simulink model "planner_contral"  (R2023b)
settings: Solver=FixedStepAuto  StartTime=0  StopTime=inf  FixedStep=0.001  RelTol=1e-3
undefined symbols (not defined in the file): aubr, c_factor, cf, cr, iniObsHeading1, iniObsHeading2, iniObsPos1, iniObsPos2, KD_PID_distance, KD_PID_speed, KI_PID_distance, KI_PID_speed, KP_PID_distance, KP_PID_speed, la, lb, LQR_K1, LQR_K2, LQR_K3, LQR_K4, m, rack_displacement, refInfo_obs1, refInfo_obs2, right_wheel_ground, rightWaypoints, tablebr, vubr, vx_break_point
libraries: Solver_SF x1
(part 8 of 8)

== matlab function planner_contral/Subsystem5/packaging ==
  data: dynamic_obs1_x input; obs_x_set_gcs output; dynamic_obs1_y input; dynamic_obs1_heading input; dynamic_obs1_speed input; dynamic_obs2_x input; dynamic_obs2_y input; dynamic_obs2_heading input; obs_y_set_gcs output; obs_velocity_set_gcs output; obs_heading_set_gcs output; dynamic_obs2_speed input; stactic_obs1_x input; stactic_obs1_y input; stactic_obs1_heading input; stactic_obs1_speed input; stactic_obs2_x input; stactic_obs2_y input; stactic_obs2_heading input; stactic_obs2_speed input
function [obs_x_set_gcs,obs_y_set_gcs,obs_velocity_set_gcs,obs_heading_set_gcs] = ...
    fcn(dynamic_obs1_x,dynamic_obs1_y,dynamic_obs1_heading,dynamic_obs1_speed,...
    dynamic_obs2_x,dynamic_obs2_y,dynamic_obs2_heading,dynamic_obs2_speed,...
    stactic_obs1_x,stactic_obs1_y,stactic_obs1_heading,stactic_obs1_speed,...
    stactic_obs2_x,stactic_obs2_y,stactic_obs2_heading,stactic_obs2_speed)
%gcs 全局坐标系global coordinate system
%该函数是感知模块，输出障碍物的位置，速度大小，速度方向与世界坐标系x轴的夹角
%输入：定位信息host_x,host_y,host_heading_xy 世界坐标系
%      障碍物在传感器坐标系下的极坐标range，theta
%      障碍物的速度大小 velocity
%      障碍物的速度方向与x轴的夹角 heading
%输出：障碍物在世界坐标系下的坐标 x y v v与x轴的夹角heading
%      注意输出的heading是障碍物的速度heading，不是障碍物的几何heading

%传感器最多输出32个障碍物信息，但是事先不知道有多少个障碍物，所以要做个缓冲

%输出初始化
obs_x_set_gcs = ones(32,1)*nan;
obs_y_set_gcs = ones(32,1)*nan;
obs_velocity_set_gcs = ones(32,1)*nan;
obs_heading_set_gcs = ones(32,1)*nan;
%传感器极坐标的角度顺时针为正，世界坐标是逆时针为正


%计算障碍物的世界坐标

% ===== 1) dynamic obstacle 1 =====
obs_x_set_gcs(1) = dynamic_obs1_x;
obs_y_set_gcs(1) = dynamic_obs1_y;
obs_heading_set_gcs(1) = dynamic_obs1_heading;
obs_velocity_set_gcs(1) = dynamic_obs1_speed;

% ===== 2) dynamic obstacle 2 =====
obs_x_set_gcs(2) = dynamic_obs2_x;
obs_y_set_gcs(2) = dynamic_obs2_y;
obs_heading_set_gcs(2) = dynamic_obs2_heading;
obs_velocity_set_gcs(2) = dynamic_obs2_speed;

% ===== 3) static obstacle 1 =====
obs_x_set_gcs(3) = stactic_obs1_x;
obs_y_set_gcs(3) = stactic_obs1_y;
obs_heading_set_gcs(3) = stactic_obs1_heading;
obs_velocity_set_gcs(3) = stactic_obs1_speed;

% ===== 4) static obstacle 2 =====
obs_x_set_gcs(4) = stactic_obs2_x;
obs_y_set_gcs(4) = stactic_obs2_y;
obs_heading_set_gcs(4) = stactic_obs2_heading;
obs_velocity_set_gcs(4) = stactic_obs2_speed;

== matlab function planner_contral/decision_planning/EMplanner/path decision task/increase DP path nodes ==
  data: dp_path_s_init input; dp_path_s_final output; dp_path_l_init input; plan_start_s input; plan_start_l input; plan_start_dl input; plan_start_ddl input; dp_path_l_final output; dp_path_dl_final output; dp_path_ddl_final output
function [dp_path_s_final,dp_path_l_final,dp_path_dl_final,dp_path_ddl_final] = ...
    fcn(dp_path_s_init,dp_path_l_init,plan_start_s,plan_start_l,plan_start_dl,plan_start_ddl)
% 该函数将增密dp_path_s,dp_path_l
% 由于事先不知道动态规划采样的行和列，也就不知道动态规划计算的曲线有多长，因此需要做缓冲
% 每1“米”采样一个点，一共采60个
ds = 1;
% 输出初始化
dp_path_s_final = ones(60,1)*nan;
dp_path_l_final = ones(60,1)*nan;
dp_path_dl_final = ones(60,1)*nan;
dp_path_ddl_final = ones(60,1)*nan;

% 设置五次多项式的起点
start_s = plan_start_s;
start_l = plan_start_l;
start_dl = plan_start_dl;
start_ddl = plan_start_ddl;

s_cur = [];
l_temp = [];
dl_temp =[];
ddl_temp = [];

for i = 1:length(dp_path_s_init)
    if dp_path_s_init(i) == -1
        break;
    end
    for j = 1:10000
        %采样s
        s_node = start_s + ds*(j - 1);
        if s_node < dp_path_s_init(i)
            s_cur = [s_cur,s_node];
        else
            break;
        end
    end
    end_s = dp_path_s_init(i);
    end_l = dp_path_l_init(i);
    end_dl = 0;
    end_ddl = 0;
    coeff = CalcQuinticCoeffient(start_l,start_dl,start_ddl,end_l,end_dl,end_ddl,start_s,end_s);
    a0 = coeff(1);
    a1 = coeff(2);
    a2 = coeff(3);
    a3 = coeff(4);
    a4 = coeff(5);
    a5 = coeff(6);
    l = a0 * ones(1,length(s_cur)) + a1 * s_cur + a2 * s_cur.^2 + a3 * s_cur.^3 +...
        a4 * s_cur.^4 + a5 * s_cur.^5;
    dl = a1 * ones(1,length(s_cur)) + 2 * a2 * s_cur + 3 * a3 * s_cur.^2 + ...
        4 * a4 * s_cur.^3 + 5 * a5 * s_cur.^4;
    ddl = 2 * a2 * ones(1,length(s_cur)) + 6 * a3 * s_cur + 12 * a4 * s_cur.^2 + ...
        20 * a5 * s_cur.^3;
    % 把 l dl ddl 的结果保存
    l_temp = [l_temp,l];
    dl_temp = [dl_temp,dl];
    ddl_temp = [ddl_temp,ddl];
    % end的值赋值给start 做下一步循环
    start_s = end_s;
    start_l = end_l;
    start_dl = end_dl;
    start_ddl = end_ddl;
    s_cur = [];
end
   for k = 1:length(l_temp)
       if k == 61
           break;
       end
       dp_path_s_final(k) = plan_start_s + ds * (k - 1);
       dp_path_l_final(k) = l_temp(k);
       dp_path_dl_final(k) = dl_temp(k);
       dp_path_ddl_final(k) = ddl_temp(k);
   end
end

function coeff = CalcQuinticCoeffient(start_l,start_dl,start_ddl,end_l,end_dl,end_ddl,start_s,end_s)
    % l = a0 + a1*s + a2*s^2 + a3*s^3 + a4*s^4 + a5*s^5
    % l' = a1 + 2 * a2 * s + 3 * a3 * s^2 + 4 * a4 * s^3 + 5 * a5 * s^4
    % l'' = 2 * a2 + 6 * a3 * s + 12 * a4 * s^2 + 20 * a5 * s^3
    start_s2 = start_s * start_s;
    start_s3 = start_s2 * start_s;
    start_s4 = start_s3 * start_s;
    start_s5 = start_s4 * start_s;
    end_s2 = end_s * end_s;
    end_s3 = end_s2 * end_s;
    end_s4 = end_s3 * end_s;
    end_s5 = end_s4 * end_s;
    A = [1,start_s, start_s2,     start_s3,     start_s4,      start_s5;
         0 1,       2 * start_s,  3 * start_s2, 4 * start_s3,  5 * start_s4;
         0 0,       2,            6 * start_s,  12 * start_s2, 20 * start_s3;
         1,end_s, end_s2,     end_s3,     end_s4,      end_s5;
         0,1,     2 * end_s,  3 * end_s2, 4 * end_s3,  5 * end_s4;
         0,0,     2,          6 * end_s,  12 * end_s2, 20 * end_s3;];
    B = [start_l;
         start_dl;
         start_ddl;
         end_l;
         end_dl;
         end_ddl;];
     coeff = A \ B;
    
end

== matlab function planner_contral/decision_planning/EMplanner/path decision task/path decision with dynamic planning(dp) ==
  data: staticobs_s_set input; dp_path_s output; staticobs_l_set input; staticobs_heading input; plan_start_s input; plan_start_l input; plan_start_dl input; plan_start_dll input; w_cost_collision input; w_cost_smooth_dl input; w_cost_smooth_ddl input; w_cost_smooth_dddl input; w_cost_ref input; row input; col input; sample_s input; sample_l input; dp_path_l output; dynamic_obs_s input; dynamic_obs_l input; dynamic_obs_heading input
function [dp_path_s,dp_path_l] = fcn(staticobs_s_set,staticobs_l_set,staticobs_heading,plan_start_s,plan_start_l,plan_start_dl,...
    plan_start_dll,w_cost_collision,w_cost_smooth_dl,w_cost_smooth_ddl,w_cost_smooth_dddl,w_cost_ref,row,col,sample_s,sample_l,dynamic_obs_s,dynamic_obs_l,dynamic_obs_heading)
%该函数为路径决策算法动态规划的主函数
% 输入：obs s l set 筛选后的障碍物sl信息
%       plan_start s l dl ddl 规划起点信息
%       w_cost_obs,w_cost_smooth_dl,w_cost_smooth_ddl,w_cost_smooth_dddl,w_cost_ref动态规划代价权重
%       row col 动态规划采样点的行数和列数(row必须是奇数，col必须是6)
%       sample_s,sample_l 采样的s l 长度
% 输出：dp_path_l,dp_path_s 动态规划的路径sl,此路径不包含规划起点  

%动态规划最优的数据结构是结构体矩阵，但是simulink不支持结构体矩阵，所以动态规划算法写的相对难以理解

%声明二维矩阵变量node_cost，node_cost(i,j)表示从起点出发，到行i列j节点的最小代价为node_cost(i,j)
node_cost = ones(row,col)*inf;%初始化为无穷大

%声明二维矩阵变量pre_node_index pre_node_index(i,j)表示从起点到行i列j的节点的最优路径中前一个节点的行号为
%pre_node_index(i,j)
%例：比如一条最优路径为 起点 -> node(1,1) -> node(2,2) -> node(3,3)
%则pre_node_index(3,3) = 2 (最优路径的前一个节点是node(2,2) 取它的行号）
%  pre_node_index(2,2) = 1 (最优路径的前一个节点是node(1,1) 取它的行号）
%  pre_node_index(1,1) = 0 (起点的行号默认是0)

% 其实pre_node_index就是当找到最小代价的路径后从终点到起点反向选择出最优路径的
%如果用结构体矩阵完全没有必要弄得这么麻烦，但是simulink不支持
pre_node_index = zeros(row,col);%初始化，所有节点的上个最优节点的行号都是0，也就是起点

%先计算从起点到第一列的cost
for i = 1:row
    node_cost(i,1) = CalcStartCost(plan_start_s,plan_start_l,plan_start_dl,...
    plan_start_dll,i,sample_s,sample_l,w_cost_collision,w_cost_smooth_dl,...
    w_cost_smooth_ddl,w_cost_smooth_dddl,w_cost_ref,staticobs_s_set,staticobs_l_set,staticobs_heading,row)+ CalcStartCost(plan_start_s,plan_start_l,plan_start_dl,...
    plan_start_dll,i,sample_s,sample_l,w_cost_collision,w_cost_smooth_dl,...
    w_cost_smooth_ddl,w_cost_smooth_dddl,w_cost_ref,dynamic_obs_s,dynamic_obs_l,dynamic_obs_heading,row);
end
% 动态规划主函数，从第二列开始
for j = 2:col
    for i = 1:row
        %计算当前node(i,j)的s l
        cur_node_s = plan_start_s + j * sample_s;
        cur_node_l = ((row + 1)/2 - i) * sample_l;
        %遍历前一列的节点
        for k = 1:row
            %计算前一列节点的s l
            pre_node_s = plan_start_s + (j - 1) * sample_s;
            pre_node_l = ((row + 1)/2 - k) * sample_l;
            cost_neighbour = CalcNeighbourCost(pre_node_s,pre_node_l,cur_node_s,cur_node_l,w_cost_collision,...
    w_cost_smooth_dl,w_cost_smooth_ddl,w_cost_smooth_dddl,w_cost_ref,staticobs_s_set,staticobs_l_set,staticobs_heading)+ CalcNeighbourCost(pre_node_s,pre_node_l,cur_node_s,cur_node_l,w_cost_collision,...
    w_cost_smooth_dl,w_cost_smooth_ddl,w_cost_smooth_dddl,w_cost_ref,dynamic_obs_s,dynamic_obs_l,dynamic_obs_heading);
            %起点到上一个节点的最小代价为node_cost(k,j-1)
            pre_min_cost = node_cost(k,j-1);
            %起点到node_cost(i,j)的最小代价 为node_cost(k,j-1)
            %再加上node(k,j-1)到node(i,j)的代价 (k = 1,2,3,4...row) 中最小的
            cost_temp = pre_min_cost + cost_neighbour;
            if cost_temp < node_cost(i,j)
                node_cost(i,j) = cost_temp;
                %把最优路径上一列节点的行号记录下来
                pre_node_index(i,j) = k;
            end
        end      
    end
end
%找到node_cost最后一列中，cost最小的，记代价最小的行号为index
index = 0;
min_cost = inf;
for i = 1:row
    if node_cost(i,end) < min_cost
        min_cost = node_cost(i,end);
        index = i;
    end
end
%动态规划最优路径初始化
dp_node_list_row = zeros(col,1);
%从后往前逆推
cur_index = index;
for i = 1:col
    %记录cur_index前面节点的行号
    pre_index = pre_node_index(cur_index,end - i + 1);
    %把cur_index放到dp_node_list_row对应的位置
    dp_node_list_row(col - i + 1) = cur_index;
    %再把pre_index 赋给 cur_index 进行下一步递推
    cur_index = pre_index;
end
% 输出初始化，由于事先不知道横纵向的采样列数，因此需要做缓冲，横纵向采样的列数不就是固定下来的吗？？？笑话
dp_path_s = ones(15,1)*-1;
dp_path_l = ones(15,1)*-1;
for i = 1:col  %最多到col，其余均为-1；
    dp_path_s(i) = plan_start_s + i * sample_s;
    dp_path_l(i) = ((row + 1) / 2 - dp_node_list_row(i)) * sample_l;
end

end
function cost = CalcNeighbourCost(pre_node_s,pre_node_l,cur_node_s,cur_node_l,w_cost_collision,...
    w_cost_smooth_dl,w_cost_smooth_ddl,w_cost_smooth_dddl,w_cost_ref,obs_s_set,obs_l_set,obs_heading_set)
% 该函数将计算相邻两个节点之间的cost
  
   start_l = pre_node_l;
    start_dl = 0;
    start_ddl = 0;
    end_l = cur_node_l;
    end_dl = 0;
    end_ddl = 0;
    start_s = pre_node_s;
    end_s = cur_node_s;
    coeff = CalcQuinticCoeffient(start_l,start_dl,start_ddl,end_l,end_dl,end_ddl,start_s,end_s);
    a0 = coeff(1);
    a1 = coeff(2);
    a2 = coeff(3);
    a3 = coeff(4);
    a4 = coeff(5);
    a5 = coeff(6);
    % 取10个点计算cost
    ds = zeros(10,1);
    l = zeros(10,1);
    dl = zeros(10,1);
    ddl = zeros(10,1);
    dddl = zeros(10,1);
    for i = 1:10
        ds(i) = start_s + (i-1)*(end_s - start_s)/10;
    end
    l = a0 * ones(10,1) + a1 * ds + a2 * ds.^2 + a3 * ds.^3 + a4 * ds.^4 + a5 * ds.^5;
    dl = a1 * ones(10,1) + 2 * a2 * ds + 3 * a3 * ds.^2 + 4 * a4 * ds.^3 + 5 * a5 * ds.^4;
    ddl = 2 * a2 * ones(10,1) + 6 * a3 * ds + 12 * a4 * ds.^2 + 20 * a5 * ds.^3;
    dddl = 6 * ones(10,1) * a3 + 24 * a4 * ds + 60 * a5 * ds.^2;
    cost_smooth = w_cost_smooth_dl * (dl' * dl) + w_cost_smooth_ddl * (ddl' * ddl) + w_cost_smooth_dddl * (dddl' * dddl);
    for i = 1:length(ddl)
        if abs(ddl(i))> 0.5 || abs(atan(dl(i))) > 0.4*pi
            cost_smooth = cost_smooth + 1e7;
            break;
        end
    end
    cost_ref = w_cost_ref * (l' * l);
%计算静态障碍物代价，实际障碍物的航向角以及
    cost_collision = 0;
    for i = 1:length(obs_s_set)
        if isnan(obs_s_set(i))
            break;
        end
     %首先对障碍物,获取障碍物的四个角点位置信息
     [s_point,l_point,l_max,l_min,s_max,s_min]=getboxpoint(obs_s_set(i),obs_l_set(i),obs_heading_set(i));
    
     %计算10个点依次到障碍物点的代价，依次计算10个点到障碍物的代价
     for j=1:length(ds)
         %获取车辆四个角点的坐标，按道理应该是如此
         %计算车辆四个角点到每一个点到障碍物角点的距离，粗略计算
         adc_front_s=ds(j)+2.5;
         adc_end_s=ds(j)-2.5;
         adc_left_l=l(j)+0.8;
         adc_right_l=l(j)-0.8;
         if(adc_left_l+0.2)<l_min||(adc_right_l-0.2)> l_max
             cost_collision=0;
             continue;
         end
         %判断当前点是否会与障碍物重叠
         if(adc_front_s<s_min)||(adc_end_s>s_max)||...
                 (adc_left_l+0.2<l_min)||((adc_right_l-0.2)> l_max)
               cost_collision=0;
         else
             cost_collision=inf;
              continue;
         end
         %判断点是否落在障碍物范围内，若落在障碍物范围内设置为无穷大
         if s_min<=ds(j)&&ds(j)<=s_max&&l_min<=l(j)&&l(j)<=l_max
              cost_collision=inf;
              continue;
         end

  %开始计算障碍物代价

        cost_collision_once = CalcObsCost(w_cost_collision,l_max,l_min,s_max,s_min,ds(j),l(j));
        cost_collision = cost_collision + cost_collision_once;
        % 判断障碍物的左右
        v1 = [ds(end);l(end)] - [ds(1);l(1)];
        v2 = [obs_s_set(i);obs_l_set(i)] - [ds(1);l(1)];
        flag = v1(1)*v2(2) - v1(2)*v2(1);
        if flag < 0 && cost_collision > 0
            cost_collision = cost_collision - 1000;
        end
    end
    end
    cost = cost_collision + cost_smooth + cost_ref;


end


function cost = CalcStartCost(begin_s,begin_l,begin_dl,begin_ddl,cur_node_row,sample_s,sample_l,w_cost_collision,...
    w_cost_smooth_dl,w_cost_smooth_ddl,w_cost_smooth_dddl,w_cost_ref,obs_s_set,obs_l_set,obs_heading,row)
    %该函数将计算起点到第一层的cost
    start_l = begin_l;
    start_dl = begin_dl;
    start_ddl = begin_ddl;
    %  . . .
    %  . . . row = 3 中间的行号 = (row + 1) /2 = 2
    %  . . .
    end_l = ((row + 1)/2 - cur_node_row)*sample_l;
    end_dl = 0;
    end_ddl = 0;
    start_s = begin_s;
    end_s = begin_s + sample_s;
    coeff = CalcQuinticCoeffient(start_l,start_dl,start_ddl,end_l,end_dl,end_ddl,start_s,end_s);
    a0 = coeff(1);
    a1 = coeff(2);
    a2 = coeff(3);
    a3 = coeff(4);
    a4 = coeff(5);
    a5 = coeff(6);
    % 取10个点计算cost
    ds = zeros(10,1);
    l = zeros(10,1);
    dl = zeros(10,1);
    ddl = zeros(10,1);
    dddl = zeros(10,1);
    for i = 1:10
        ds(i) = start_s + (i-1)*sample_s/10;
    end
    l = a0 * ones(10,1) + a1 * ds + a2 * ds.^2 + a3 * ds.^3 + a4 * ds.^4 + a5 * ds.^5;
    dl = a1 * ones(10,1) + 2 * a2 * ds + 3 * a3 * ds.^2 + 4 * a4 * ds.^3 + 5 * a5 * ds.^4;
    ddl = 2 * a2 * ones(10,1) + 6 * a3 * ds + 12 * a4 * ds.^2 + 20 * a5 * ds.^3;
    dddl = 6 * ones(10,1) * a3 + 24 * a4 * ds + 60 * a5 * ds.^2;
    cost_smooth = w_cost_smooth_dl * (dl' * dl) + w_cost_smooth_ddl * (ddl' * ddl) + w_cost_smooth_dddl * (dddl' * dddl);
    for i = 1:length(dl)
        if abs(ddl(i))> 0.5 || abs(atan(dl(i))) > 0.4*pi
            cost_smooth = cost_smooth + 1e7;
            break;
        end
    end
    cost_ref = w_cost_ref * (l' * l);
    cost_collision = 0;
    for i = 1:length(obs_s_set)
        if isnan(obs_s_set(i))
            break;
        end
        %首先对障碍物四个角点坐标
      [s_point,l_point,l_max,l_min,s_max,s_min]=getboxpoint(obs_s_set(i),obs_l_set(i),obs_heading(i));
     %计算10个点依次到障碍物点的代价，依次计算10个点到障碍物的代价
     for j=1:length(ds)
         %计算每一个点到障碍物的距离
         adc_front_s=ds(j)+2.5;
         adc_end_s=ds(j)-2.5;
         adc_left_l=l(j)+0.8;
         adc_right_l=l(j)-0.8;
   
         if(adc_left_l+0.2)<l_min||(adc_right_l-0.2)> l_max
             cost_collision=0;
              continue;
         end
         %判断当前点是否会与障碍物重叠
          if(adc_front_s<s_min)||(adc_end_s>s_max)||...
                 (adc_left_l+0.2<l_min)||((adc_right_l-0.2)> l_max) 
              cost_collision=0;
          else
             cost_collision=inf;
              continue;
         end
         if s_min<=ds(j)&&ds(j)<=s_max&&l_min<=l(j)&&l(j)<=l_max
              cost_collision=inf;
              continue;
         end

        cost_collision_once = CalcObsCost(w_cost_collision,l_max,l_min,s_max,s_min,ds(j),l(j));
        cost_collision = cost_collision + cost_collision_once;
        % 判断障碍物的左右
        v1 = [ds(end);l(end)] - [ds(1);l(1)];
        v2 = [obs_s_set(i);obs_l_set(i)] - [ds(1);l(1)];
        flag = v1(1)*v2(2) - v1(2)*v2(1);
        if flag < 0 && cost_collision > 0
            cost_collision = cost_collision - 1000;
        end
      end

    end
    
    cost = cost_collision + cost_smooth + cost_ref;
      
    end
%计算静态障碍物代价
function obs_cost = CalcObsCost(w_cost_collision,l_max,l_min,s_max,s_min,cur_ds,cur_l)
%该函数将计算障碍物的距离代价，计算该点到四个角点的代价函数
%横向代价

   delta_l=abs(cur_l-(l_min+l_max)/2     );
   cost_l=w_cost_collision*(1/(1+exp(0.5-delta_l)));

%纵向代价
   delta_s=abs(cur_ds-(s_min+s_max)/2     );
   cost_s=w_cost_collision*(1/(1+exp(0.5-delta_s)));
    obs_cost =cost_l+cost_s;
end



function coeff = CalcQuinticCoeffient(start_l,start_dl,start_ddl,end_l,end_dl,end_ddl,start_s,end_s)
    % l = a0 + a1*s + a2*s^2 + a3*s^3 + a4*s^4 + a5*s^5
    % l' = a1 + 2 * a2 * s + 3 * a3 * s^2 + 4 * a4 * s^3 + 5 * a5 * s^4
    % l'' = 2 * a2 + 6 * a3 * s + 12 * a4 * s^2 + 20 * a5 * s^3
    start_s2 = start_s * start_s;
    start_s3 = start_s2 * start_s;
    start_s4 = start_s3 * start_s;
    start_s5 = start_s4 * start_s;
    end_s2 = end_s * end_s;
    end_s3 = end_s2 * end_s;
    end_s4 = end_s3 * end_s;
    end_s5 = end_s4 * end_s;
    A = [1,start_s, start_s2,     start_s3,     start_s4,      start_s5;
         0 1,       2 * start_s,  3 * start_s2, 4 * start_s3,  5 * start_s4;
         0 0,       2,            6 * start_s,  12 * start_s2, 20 * start_s3;
         1,end_s, end_s2,     end_s3,     end_s4,      end_s5;
         0,1,     2 * end_s,  3 * end_s2, 4 * end_s3,  5 * end_s4;
         0,0,     2,          6 * end_s,  12 * end_s2, 20 * end_s3;];
    B = [start_l;
         start_dl;
         start_ddl;
         end_l;
         end_dl;
         end_ddl;];
     coeff = A \ B;
    
end
function [s_set,l_set,l_max,l_min,s_max,s_min]=getboxpoint(obs_s,obs_l,obs_heading)
%获取车辆后轴中心点
obs_length=5;
obs_width=2;
    l_set=zeros(4,1);
    s_set=zeros(4,1);
    rear_s = obs_s;
    rear_l = obs_l;
%计算前轴中心点
    front_s=rear_s+obs_length*cos(obs_heading);
    front_l=rear_l+obs_length*sin(obs_heading);
 %计算四个角点的的l及s
    l_ringht_upper=front_l+obs_width/2*cos(obs_heading);
    s_ringht_upper=front_s-obs_width/2*sin(obs_heading);

    l_right_low=front_l-obs_width/2*cos(obs_heading);
    s_right_low=front_s+obs_width/2*sin(obs_heading);

    l_left_upper=rear_l+obs_width/2*cos(obs_heading);
    s_left_upper=rear_s-obs_width/2*sin(obs_heading);

    l_left_low=rear_l-obs_width/2*cos(obs_heading);
    s_left_low= rear_s+obs_width/2*sin(obs_heading);
 

    l_set(1)= l_ringht_upper;
    l_set(2)=l_right_low;
    l_set(3)=l_left_upper;
    l_set(4)=l_left_low;
    s_set(1)= s_ringht_upper;
    s_set(2)=s_right_low;
    s_set(3)=s_left_upper;
    s_set(4)=s_left_low;
    l_max=max(l_set);
    l_min=min(l_set);
    s_max=max(s_set);
    s_min=min(s_set);

end
